simulink model "HANcoder_E407_SMV_program"  (R2018a)
settings: Solver=FixedStepDiscrete  StartTime=0.0  StopTime=1  FixedStep=0.01  RelTol=1e-3
PreLoadFcn:
  | librarySetup
  | eval([bdroot,'_startup']) %Calling [modelName]_startup.m
values from neighbouring files (symbols this model uses):
  Speed = [0.4; 0.4; 0.4; 0.4; 0.4; 0.4; 0.4; 0.4; 0.4; 0.4;0]    [Xbee_Track_Presentation.m]
undefined symbols (not defined in the file or in its folder): A0, A1, A2, A3, b, CON2, CON3, CON4, D13, D4, D5, drivemode, L_D1, L_D2, manual_xbee_switch, Steering_angle, steermode
libraries: HANcoder_STM32_Target x38, simulink_extras x11, simulink x7
(part 3 of 3)

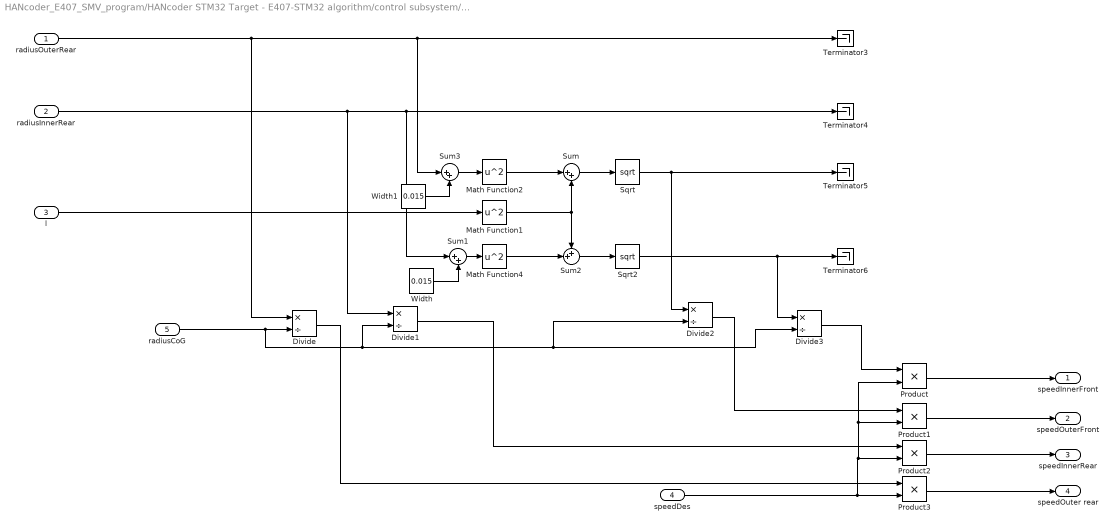
== system HANcoder_E407_SMV_program/HANcoder STM32 Target - E407-STM32 algorithm/control subsystem/2 wheel steering/SpeedAngleCalculator1/Speed calculator ==
  radiusOuterRear : Inport
  radiusInnerRear : Inport  Port=2
  l : Inport  Port=3
  speedDes : Inport  Port=4
  radiusCoG : Inport  Port=5
  Divide{,1..3} (4 alike) : Product  Inputs=*/
  Math Function1 : Math  Operator=square  SaturateOnIntegerOverflow=on
  Math Function2 : Math  Operator=square  SaturateOnIntegerOverflow=on
  Math Function4 : Math  Operator=square  SaturateOnIntegerOverflow=on
  Product{,1..3} (4 alike) : Product
  Sqrt : Sqrt  SaturateOnIntegerOverflow=on
  Sqrt2 : Sqrt  SaturateOnIntegerOverflow=on
  Sum : Sum  Inputs=|++
  Sum1 : Sum  Inputs=|++
  Sum2 : Sum  Inputs=++|
  Sum3 : Sum  Inputs=|++
  Terminator{3..6} (4 alike) : Terminator
  Width : Constant  Value=0.015
  Width1 : Constant  Value=0.015
  speedInnerFront : Outport
  speedOuterFront : Outport  Port=2
  speedInnerRear : Outport  Port=3
  speedOuter rear : Outport  Port=4
  wires:
  Math Function2/1 -> Sum/1
  Sum/1 -> Sqrt/1
  Sum2/1 -> Sqrt2/1
  Math Function1/1 -> Sum2/1, Sum/2
  Sqrt2/1 -> Divide3/1, Terminator6/1
  radiusInnerRear/1 -> Divide1/1, Sum1/1, Terminator4/1
  Sqrt/1 -> Divide2/1, Terminator5/1
  Math Function4/1 -> Sum2/2
  l/1 -> Math Function1/1
  radiusCoG/1 -> Divide3/2, Divide2/2, Divide1/2, Divide/2
  speedDes/1 -> Product/2, Product1/2, Product2/2, Product3/2
  Divide3/1 -> Product/1
  Divide2/1 -> Product1/1
  Divide1/1 -> Product2/1
  Divide/1 -> Product3/1
  Product/1 -> speedInnerFront/1
  Product1/1 -> speedOuterFront/1
  Product2/1 -> speedInnerRear/1
  Product3/1 -> speedOuter rear/1
  Width/1 -> Sum1/2
  Width1/1 -> Sum3/2
  Sum3/1 -> Math Function2/1
  radiusOuterRear/1 -> Divide/1, Sum3/1, Terminator3/1
  Sum1/1 -> Math Function4/1

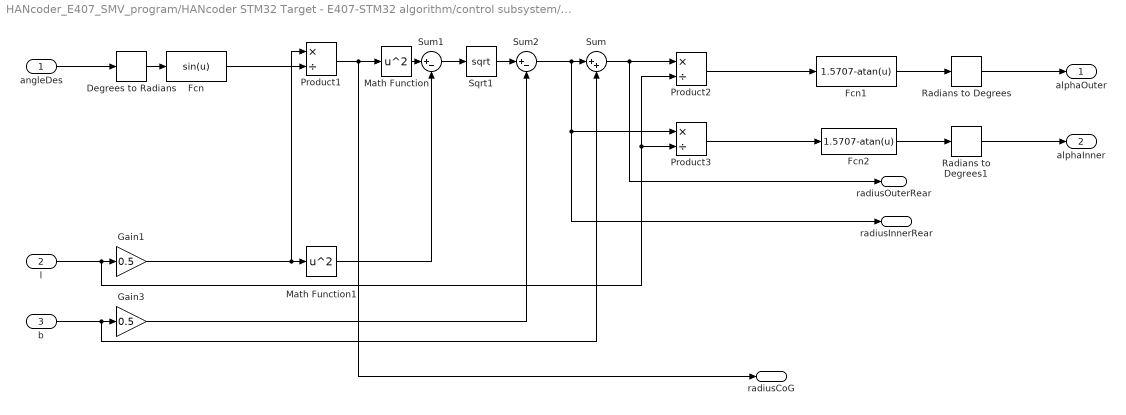
== system HANcoder_E407_SMV_program/HANcoder STM32 Target - E407-STM32 algorithm/control subsystem/2 wheel steering/SpeedAngleCalculator1/Steerangle calculator ==
  angleDes : Inport
  l : Inport  Port=2
  b : Inport  Port=3
  Degrees to Radians : simulink_extras/Transformations/Degrees to Radians
  Fcn : Fcn  Expr=sin(u)
  Fcn1 : Fcn  Expr=1.5707-atan(u)
  Fcn2 : Fcn  Expr=1.5707-atan(u)
  Gain1 : Gain  Gain=0.5
  Gain3 : Gain  Gain=0.5
  Math Function : Math  Operator=square  SaturateOnIntegerOverflow=on
  Math Function1 : Math  Operator=square  SaturateOnIntegerOverflow=on
  Product1 : Product  Inputs=*/
  Product2 : Product  Inputs=*/
  Product3 : Product  Inputs=*/
  Radians to Degrees : simulink_extras/Transformations/Radians to Degrees
  Radians to Degrees1 : simulink_extras/Transformations/Radians to Degrees
  Sqrt1 : Sqrt  SaturateOnIntegerOverflow=on
  Sum : Sum  Inputs=|++
  Sum1 : Sum  Inputs=|+-
  Sum2 : Sum  Inputs=|+-
  alphaOuter : Outport
  alphaInner : Outport  Port=2
  radiusOuterRear : Outport  Port=3
  radiusInnerRear : Outport  Port=4
  radiusCoG : Outport  Port=5
  wires:
  Fcn2/1 -> Radians to Degrees1/1
  Product1/1 -> radiusCoG/1, Math Function/1
  Gain1/1 -> Math Function1/1, Product1/1
  Sum2/1 -> Product3/1, radiusInnerRear/1, Sum/1
  Sqrt1/1 -> Sum2/1
  Product2/1 -> Fcn1/1
  Math Function/1 -> Sum1/1
  b/1 -> Sum/2, Gain3/1
  Math Function1/1 -> Sum1/2
  Fcn1/1 -> Radians to Degrees/1
  Sum1/1 -> Sqrt1/1
  Gain3/1 -> Sum2/2
  l/1 -> Product3/2, Product2/2, Gain1/1
  Sum/1 -> radiusOuterRear/1, Product2/1
  Degrees to Radians/1 -> Fcn/1
  Radians to Degrees/1 -> alphaOuter/1
  Fcn/1 -> Product1/2
  Product3/1 -> Fcn2/1
  angleDes/1 -> Degrees to Radians/1
  Radians to Degrees1/1 -> alphaInner/1

== system HANcoder_E407_SMV_program/HANcoder STM32 Target - E407-STM32 algorithm/control subsystem/4 wheel steering/Subsystem1/Angle inner wheels ==
  l : Inport
  Rzw : Inport  Port=2
  b : Inport  Port=3
  Fcn1 : Fcn  Expr=atan(u)
  Gain1 : Gain  Gain=1/2
  Gain2 : Gain  Gain=1/2
  Product1 : Product  Inputs=*/
  Radians to Degrees1 : simulink_extras/Transformations/Radians to Degrees
  Sum1 : Sum  Inputs=|+-
  AlphaInner : Outport
  wires:
  Fcn1/1 -> Radians to Degrees1/1
  Product1/1 -> Fcn1/1
  Radians to Degrees1/1 -> AlphaInner/1
  Sum1/1 -> Product1/2
  l/1 -> Gain1/1
  b/1 -> Gain2/1
  Rzw/1 -> Sum1/1
  Gain2/1 -> Sum1/2
  Gain1/1 -> Product1/1

== system HANcoder_E407_SMV_program/HANcoder STM32 Target - E407-STM32 algorithm/control subsystem/4 wheel steering/Subsystem1/Angle outer wheels ==
  l : Inport
  Rzw : Inport  Port=2
  b : Inport  Port=3
  Fcn : Fcn  Expr=atan(u)
  Gain1 : Gain  Gain=1/2
  Gain2 : Gain  Gain=1/2
  Product : Product  Inputs=*/
  Radians to Degrees : simulink_extras/Transformations/Radians to Degrees
  Sum : Sum  Inputs=|++
  AlphaOuter : Outport
  wires:
  b/1 -> Gain2/1
  Rzw/1 -> Sum/1
  l/1 -> Gain1/1
  Fcn/1 -> Radians to Degrees/1
  Radians to Degrees/1 -> AlphaOuter/1
  Sum/1 -> Product/2
  Product/1 -> Fcn/1
  Gain2/1 -> Sum/2
  Gain1/1 -> Product/1

== system HANcoder_E407_SMV_program/HANcoder STM32 Target - E407-STM32 algorithm/control subsystem/4 wheel steering/Subsystem1/Angle to radius CoG ==
  l : Inport
  "angleDes " : Inport  Port=2
  Degrees to Radians : simulink_extras/Transformations/Degrees to Radians
  Fcn1 : Fcn  Expr=sin(u)
  Gain1 : Gain  Gain=1/2
  Product1 : Product  Inputs=*/
  Rzw : Outport
  wires:
  Degrees to Radians/1 -> Fcn1/1
  Product1/1 -> Rzw/1
  l/1 -> Gain1/1
  "angleDes "/1 -> Degrees to Radians/1
  Fcn1/1 -> Product1/2
  Gain1/1 -> Product1/1

== system HANcoder_E407_SMV_program/HANcoder STM32 Target - E407-STM32 algorithm/control subsystem/4 wheel steering/Subsystem1/radius inner wheel ==
  l : Inport
  b : Inport  Port=2
  Rzw : Inport  Port=3
  Gain : Gain  Gain=1/2
  Gain1 : Gain  Gain=1/2
  Math Function : Math  Operator=square  SaturateOnIntegerOverflow=on
  Math Function1 : Math  Operator=square  SaturateOnIntegerOverflow=on
  Sqrt : Sqrt  SaturateOnIntegerOverflow=on
  Sum : Sum  Inputs=|++
  Sum1 : Sum  Inputs=|-+
  radiusInner : Outport
  wires:
  Gain1/1 -> Sum1/1
  Gain/1 -> Math Function/1
  Math Function1/1 -> Sum/2
  l/1 -> Gain/1
  Sum/1 -> Sqrt/1
  Math Function/1 -> Sum/1
  Rzw/1 -> Sum1/2
  b/1 -> Gain1/1
  Sqrt/1 -> radiusInner/1
  Sum1/1 -> Math Function1/1

== system HANcoder_E407_SMV_program/HANcoder STM32 Target - E407-STM32 algorithm/control subsystem/4 wheel steering/Subsystem1/radius outer wheel ==
  l : Inport
  b : Inport  Port=2
  Rzw : Inport  Port=3
  Gain : Gain  Gain=1/2
  Gain1 : Gain  Gain=1/2
  Math Function : Math  Operator=square  SaturateOnIntegerOverflow=on
  Math Function1 : Math  Operator=square  SaturateOnIntegerOverflow=on
  Sqrt : Sqrt  SaturateOnIntegerOverflow=on
  Sum : Sum  Inputs=|++
  Sum1 : Sum  Inputs=|++
  radiusOuter : Outport
  wires:
  Sum1/1 -> Math Function1/1
  Sqrt/1 -> radiusOuter/1
  b/1 -> Gain1/1
  Rzw/1 -> Sum1/2
  Math Function/1 -> Sum/1
  Sum/1 -> Sqrt/1
  l/1 -> Gain/1
  Math Function1/1 -> Sum/2
  Gain/1 -> Math Function/1
  Gain1/1 -> Sum1/1

== system HANcoder_E407_SMV_program/HANcoder STM32 Target - E407-STM32 algorithm/control subsystem/4 wheel steering/Subsystem1/speed calculator ==
  radiusOuter : Inport
  Rzw : Inport  Port=2
  radiusInner : Inport  Port=3
  speed : Inport  Port=4
  Product : Product  Inputs=*/
  Product1 : Product  Inputs=*/
  Product2 : Product
  Product3 : Product
  speedInner : Outport
  speedOuter : Outport  Port=2
  wires:
  Product1/1 -> Product3/2
  Product/1 -> Product2/1
  speed/1 -> Product3/1, Product2/2
  Rzw/1 -> Product1/2, Product/2
  radiusOuter/1 -> Product/1
  radiusInner/1 -> Product1/1
  Product3/1 -> speedInner/1
  Product2/1 -> speedOuter/1

== system HANcoder_E407_SMV_program/HANcoder STM32 Target - E407-STM32 algorithm/Xbee controll/Check received data/Check received data/Check next 3 bytes and send via CAN/Enabled Subsystem ==
  In1 : Inport
  In2 : Inport  Port=2
  Enable : EnablePort
  Out1 : Outport
  Out2 : Outport  Port=2
  wires:
  In2/1 -> Out2/1
  In1/1 -> Out1/1

== system HANcoder_E407_SMV_program/HANcoder STM32 Target - E407-STM32 algorithm/Xbee controll/Check received data/Check received data/Check next 3 bytes and send via CAN/UART stop ==
  Level-2 M-file S-Function : M-S-Function  FunctionName=sfcn_uart_receive  Parameters=tsamp
  Term1 : Terminator
  Out1 : Outport
  wires:
  Level-2 M-file S-Function/1 -> Out1/1
  Level-2 M-file S-Function/2 -> Term1/1

== system HANcoder_E407_SMV_program/HANcoder STM32 Target - E407-STM32 algorithm/Xbee controll/Check received data/Check received data/Check next 3 bytes and send via CAN/UART value1 ==
  Level-2 M-file S-Function : M-S-Function  FunctionName=sfcn_uart_receive  Parameters=tsamp
  Term1 : Terminator
  Out1 : Outport
  wires:
  Level-2 M-file S-Function/1 -> Out1/1
  Level-2 M-file S-Function/2 -> Term1/1

== system HANcoder_E407_SMV_program/HANcoder STM32 Target - E407-STM32 algorithm/Xbee controll/Check received data/Check received data/Check next 3 bytes and send via CAN/UART value2 ==
  Level-2 M-file S-Function : M-S-Function  FunctionName=sfcn_uart_receive  Parameters=tsamp
  Term1 : Terminator
  Out1 : Outport
  wires:
  Level-2 M-file S-Function/2 -> Term1/1
  Level-2 M-file S-Function/1 -> Out1/1
